simulink model "differential"  (Simulink 7.9)
settings: Solver=ode45  StartTime=0.0  StopTime=10.0  RelTol=1e-3
settings Model: Creator=prakrit  LastModifiedBy=prakrit

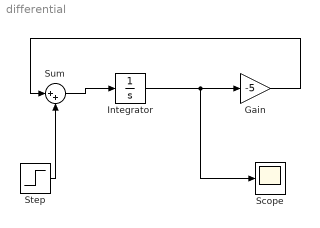
== system differential ==
  Gain : Gain  Gain=-5
  Integrator : Integrator  InitialCondition=-2
  Scope : Scope
  Step : Step  SampleTime=0
  Sum : Sum  Inputs=|++
  wires:
  Sum/1 -> Integrator/1
  Integrator/1 -> Gain/1, Scope/1
  Gain/1 -> Sum/1
  Step/1 -> Sum/2
